simulink model "zad_no_6_a"  (R2017b)
settings: Solver=VariableStepAuto  StartTime=0.0  StopTime=6  RelTol=1e-3
undefined symbols (not defined in the file): K, Tp
settings Model: Creator=micha  LastModifiedBy=micha

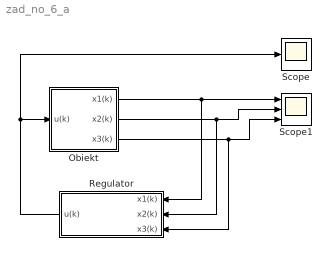
== system zad_no_6_a ==
  Obiekt : Subsystem
  Regulator : Subsystem
  Scope : Scope
  Scope1 : Scope  NumInputPorts=3
  wires:
  Regulator/1(u(k)) -> Obiekt/1(u(k)), Scope/1
  Obiekt/1(x1(k)) -> Scope1/1, Regulator/1("x1(k) ")
  Obiekt/3("x3(k) ") -> Scope1/3, Regulator/3("x3(k) ")
  Obiekt/2("x2(k) ") -> Regulator/2(x2(k)), Scope1/2

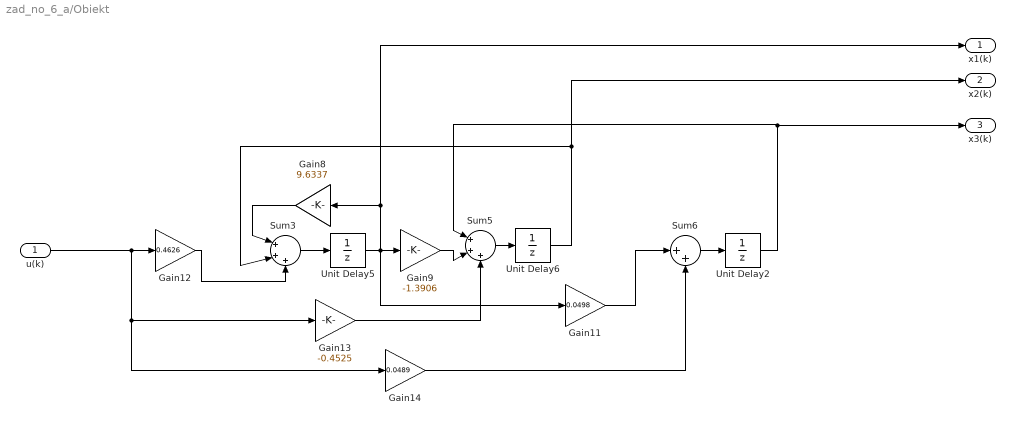
== system zad_no_6_a/Obiekt ==
  u(k) : Inport
  Gain11 : Gain  Gain=0.0498  ParamDataTypeStr=double
  Gain12 : Gain  Gain=0.4626  ParamDataTypeStr=double
  Gain13 : Gain  Gain=-0.4525  ParamDataTypeStr=double
  Gain14 : Gain  Gain=0.0489  ParamDataTypeStr=double
  Gain8 : Gain  Gain=9.6337  ParamDataTypeStr=double
  Gain9 : Gain  Gain=-1.3906  ParamDataTypeStr=double
  Sum3 : Sum  Inputs=|+++
  Sum5 : Sum  Inputs=|+++
  Sum6 : Sum  Inputs=|++
  Unit Delay2 : UnitDelay  InitialCondition=1  SampleTime=Tp
  Unit Delay5 : UnitDelay  InitialCondition=3  SampleTime=Tp
  Unit Delay6 : UnitDelay  InitialCondition=2  SampleTime=Tp
  x1(k) : Outport
  "x2(k) " : Outport  Port=2
  "x3(k) " : Outport  Port=3
  wires:
  Unit Delay6/1 -> "x2(k) "/1, Sum3/2
  Gain14/1 -> Sum6/2
  Unit Delay2/1 -> "x3(k) "/1, Sum5/1
  Unit Delay5/1 -> Gain11/1, x1(k)/1, Gain8/1, Gain9/1
  Gain13/1 -> Sum5/3
  Gain9/1 -> Sum5/2
  Gain12/1 -> Sum3/3
  Sum5/1 -> Unit Delay6/1
  Sum3/1 -> Unit Delay5/1
  Gain11/1 -> Sum6/1
  Gain8/1 -> Sum3/1
  Sum6/1 -> Unit Delay2/1
  u(k)/1 -> Gain12/1, Gain13/1, Gain14/1

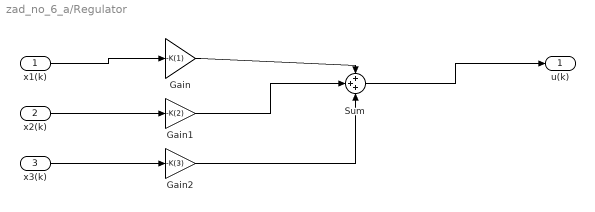
== system zad_no_6_a/Regulator ==
  "x1(k) " : Inport
  x2(k) : Inport  Port=2
  "x3(k) " : Inport  Port=3
  Gain : Gain  Gain=-K(1)
  Gain1 : Gain  Gain=-K(2)
  Gain2 : Gain  Gain=-K(3)
  Sum : Sum  Inputs=3
  u(k) : Outport
  wires:
  "x1(k) "/1 -> Gain/1
  x2(k)/1 -> Gain1/1
  "x3(k) "/1 -> Gain2/1
  Gain/1 -> Sum/1
  Gain1/1 -> Sum/2
  Gain2/1 -> Sum/3
  Sum/1 -> u(k)/1
